simulink subsystem "PieroAdry_MODEL"  (R2023b)
settings: Solver=VariableStepAuto  StartTime=0.0  StopTime=10.0  RelTol=1e-3
settings Model: Creator=adria  LastModifiedBy=adria

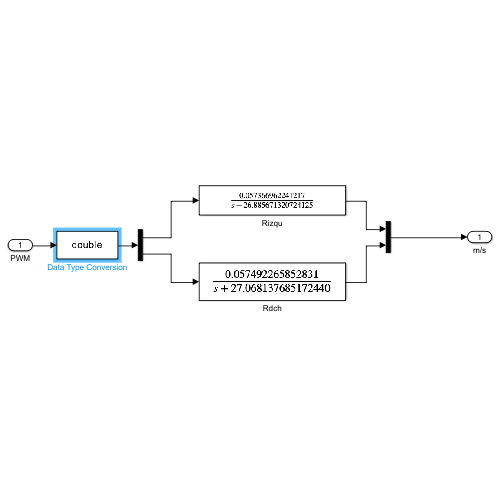
[thumbnail: Simulink's stored preview of the top-level diagram]
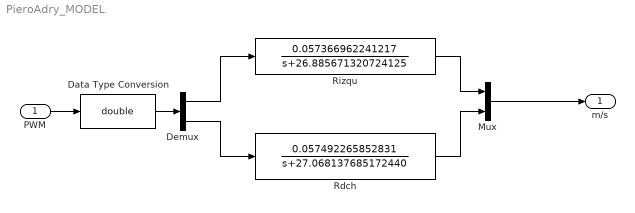
== system PieroAdry_MODEL ==
  PWM : Inport
  Data Type Conversion : DataTypeConversion  OutDataTypeStr=double  SaturateOnIntegerOverflow=off  RndMeth=Floor
  Demux : Demux  Outputs=2
  Mux : Mux  Inputs=2
  Rdch : TransferFcn  Numerator=[0.057492265852831]  Denominator=[1,27.068137685172440]
  Rizqu : TransferFcn  Numerator=[0.057366962241217]  Denominator=[1,26.885671320724125]
  m/s : Outport
  wires:
  Rizqu/1 -> Mux/1
  PWM/1 -> Data Type Conversion/1
  Demux/1 -> Rizqu/1
  Demux/2 -> Rdch/1
  Mux/1 -> m/s/1
  Rdch/1 -> Mux/2
  Data Type Conversion/1 -> Demux/1
